simulink model "nonlinear_model"  (R2020a)
settings: Solver=ode45  StartTime=0.0  StopTime=simulation_time  FixedStep=sample_time  RelTol=1e-3
values from neighbouring files (symbols this model uses):
  K = lqr(A, B, Q, R)    [lab06.m]
  sample_time = 0.03    [lab06.m]
  x0 = [0; 0; deg2rad(2); 0]    [lab06.m]
settings Model: Creator=donelp  LastModifiedBy=donelp
settings DataIOCC: SaveOutput=off  SignalLogging=off  DSMLogging=off  SaveTime=off  ReturnWorkspaceOutputs=off

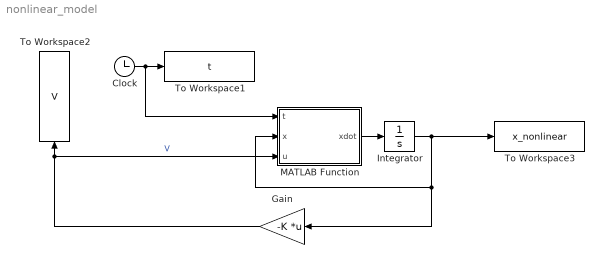
== system nonlinear_model ==
  Clock : Clock
  Gain : Gain  Gain=-K  Multiplication=Matrix(K*u)
  Integrator : Integrator  InitialCondition=x0
  MATLAB Function : MATLAB Function  TreatAsAtomicUnit=on
  To Workspace1 : ToWorkspace  VariableName=t  SampleTime=sample_time
      settings: Save2DSignal=2-D array (concatenate along first dimension)
  To Workspace2 : ToWorkspace  VariableName=V  SampleTime=sample_time
      settings: Save2DSignal=2-D array (concatenate along first dimension)
  To Workspace3 : ToWorkspace  VariableName=x_nonlinear  SampleTime=sample_time
      settings: Save2DSignal=2-D array (concatenate along first dimension)
  wires:
  Gain/1 -> MATLAB Function/3(u), To Workspace2/1  "V"
  Clock/1 -> MATLAB Function/1(t), To Workspace1/1
  MATLAB Function/1(xdot) -> Integrator/1
  Integrator/1 -> To Workspace3/1, Gain/1, MATLAB Function/2(x)

== matlab function nonlinear_model/MATLAB Function ==
  data: t input; x input; u input; xdot output
function xdot = balance_ode(t, x, u)
xdot = balance_ode(t, x, u);
